simulink model "ControlWillyBAlut"  (R2021b)
settings: Solver=FixedStepAuto  StartTime=0.0  StopTime=10.0  RelTol=1e-3  EnableMultiTasking=on
settings Model: ExtModeTrigDuration=2  Creator=yo  LastModifiedBy=yo
settings OptimizationCC: EnhancedBackFolding=on  PassReuseOutputArgsAs=Individual arguments  ZeroExternalMemoryAtStartup=off  ZeroInternalMemoryAtStartup=off  MaxStackSize=64  OptimizeBlockOrder=speed  DifferentSizesBufferReuse=on  OptimizationCustomize=off  EfficientTunableParamExpr=on
settings DebuggingCC: ParameterTunabilityLossMsg=error
settings HardwareCC: ProdBitPerInt=16  ProdBitPerPointer=16  ProdBitPerSizeT=16  ProdBitPerPtrDiffT=16  ProdLargestAtomicFloat=None  ProdWordSize=8  ProdHWDeviceType=Atmel->AVR  UseEmbeddedCoderFeatures=off  UseSimulinkCoderFeatures=off
settings SFSimCC: MATLABDynamicMemAlloc=off
settings RTWCC: Description=Embedded Coder  SystemTargetFile=ert.tlc  HardwareBoard=Arduino Mega 2560  TemplateMakefile=ert_default_tmf  Toolchain=Arduino AVR  BuildConfiguration=Faster Runs
settings CodeAppCC: ForceParamTrailComments=on  IgnoreCustomStorageClasses=off  OperatorAnnotations=on  SimulinkDataObjDesc=on  SFDataObjDesc=on  InsertBlockDesc=on
settings ERTTargetCC: SupportContinuousTime=on  SupportNonInlinedSFcns=on  SupportVariableSizeSignals=on  ExtModeTransport=3  ExtModeStaticAlloc=on  ExtModeStaticAllocSize=2048  ExtModeMexFile=ext_xcp  ExtModeIntrfLevel=Level2 - Open

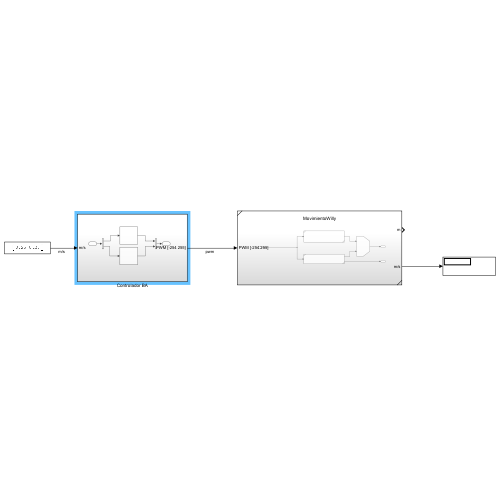
[thumbnail: Simulink's stored preview of the top-level diagram]
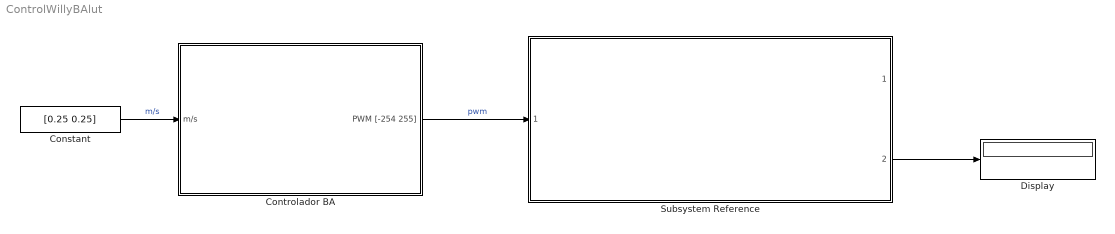
== system ControlWillyBAlut ==
  Constant : Constant  Value=[0.25 0.25]  SampleTime=0.01
  Controlador BA : Subsystem
  Display : Display
  Subsystem Reference : Subsystem  ReferencedSubsystem=MovimientoWilly
  wires:
  Controlador BA/1(PWM [-254 255]) -> Subsystem Reference/1  "pwm"
  Subsystem Reference/2 -> Display/1
  Constant/1 -> Controlador BA/1(m/s)  "m/s"

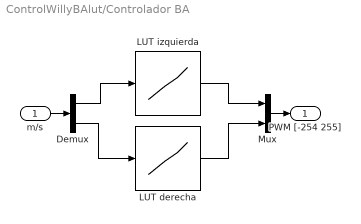
== system ControlWillyBAlut/Controlador BA ==
  m/s : Inport
  Demux : Demux  Outputs=2
  LUT derecha : Lookup_n-D  NumberOfTableDimensions=1  BreakpointsForDimension1=|  Table=|  InternalRulePriority=Speed  RndMeth=Simplest  InputSameDT=on
      BreakpointsForDimension1=|
      | [-0.598495483398438
      | -0.488235473632813
      | -0.393768310546875
      | -0.267761230468750
      | -0.126007080078125
      | 0
      | 0.157501220703125
      | 0.267730712890625
      | 0.393737792968750
      | 0.519760131835938
      | 0.614257812500000]
      Table=|
      | [-255
      | -204
      | -153
      | -102
      | -51
      | 0
      | 51.0000076293945
      | 102
      | 153
      | 204
      | 255]
  LUT izquierda : Lookup_n-D  NumberOfTableDimensions=1  BreakpointsForDimension1=|  Table=|  InternalRulePriority=Speed  RndMeth=Simplest  InputSameDT=on
      BreakpointsForDimension1=|
      | [-0.630004882812500
      | -0.519760131835938
      | -0.393737792968750
      | -0.267730712890625
      | -0.126007080078125
      | 0
      | 0.141754150390625
      | 0.267730712890625
      | 0.409515380859375
      | 0.519744873046875
      | 0.598495483398438]
      Table=|
      | [-255
      | -204
      | -153
      | -102
      | -51
      | 0
      | 51.0000076293945
      | 102
      | 153
      | 204
      | 255]
  Mux : Mux  Inputs=2
  PWM [-254 255] : Outport
  wires:
  LUT izquierda/1 -> Mux/1
  Demux/1 -> LUT izquierda/1
  Mux/1 -> PWM [-254 255]/1
  Demux/2 -> LUT derecha/1
  m/s/1 -> Demux/1
  LUT derecha/1 -> Mux/2
